simulink model "ReservoirMPC"  (R2023a)
settings: Solver=VariableStepAuto  StartTime=0.0  StopTime=100.0  RelTol=1e-3
libraries: mpclib x1
settings Model: Creator=The MathWorks, Inc.  LastModifiedBy=The MathWorks, Inc.
settings DebuggingCC: UnconnectedInputMsg=warning  UnconnectedOutputMsg=warning  UnconnectedLineMsg=warning
settings ModelReferenceCC: EnableRefExpFcnMdlSchedulingChecks=on
settings RTWCC: DLArmComputeVersion=19.05

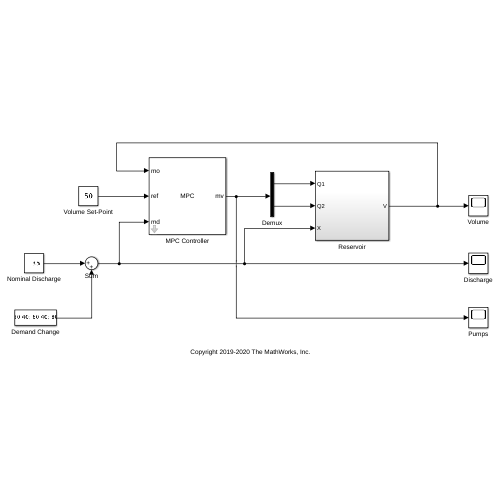
[thumbnail: Simulink's stored preview of the top-level diagram]
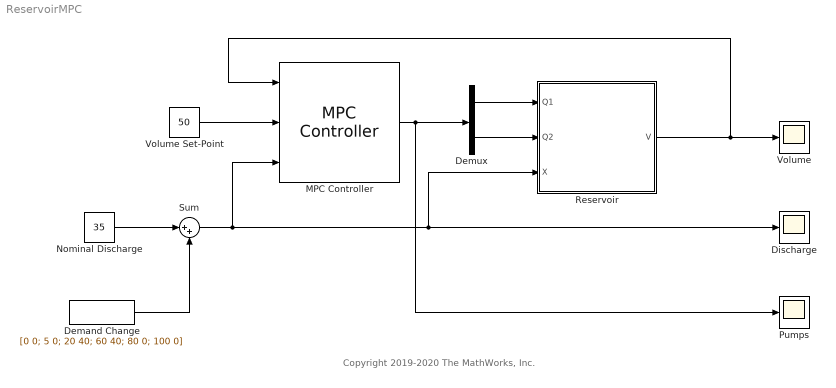
== system ReservoirMPC ==
  note: Copyright 2019-2020 The MathWorks, Inc.
  Demand Change : FromWorkspace  VariableName=[0 0; 5 0; 20 40; 60 40; 80 0; 100 0]
  Demux : Demux  Outputs=2
  Discharge : Scope
  MPC Controller : mpclib/MPC Controller  SCDEnableBlockLinearizationSpecification=on  mpcobj=mpcobj  is_multiple=0  enable_value=0  return_u0=off  updateMPCinCallerWorkspace=on  md_inport=on  mv_inport=off  uref_inport=off  return_cost=off  return_mvseq=off  return_qpstatus=off  return_xseq=off  return_state=off  return_ovseq=off  state_inport=off  umin_inport=off  umax_inport=off  ymin_inport=off  ymax_inport=off  cc_inport=off  ywt_inport=off  uwt_inport=off  duwt_inport=off  rhoeps_inport=off  pm_inport=off  MaximumP=10  HorizonChoice=FixedHorizon  n_ts=1  n_p=10  n_mv=2  n_md=1  n_ud=0  n_mo=1  n_uo=0  BlockDataType=double  SampleTimeInherited=off  switch_inport=off
  Nominal Discharge : Constant  Value=35
  Pumps : Scope
  Reservoir : Subsystem
  Sum : Sum  Inputs=|++
  Volume : Scope
  Volume Set-Point : Constant  Value=50
  wires:
  Reservoir/1(V) -> MPC Controller/1, Volume/1
  Demux/1 -> Reservoir/1(Q1)
  Demux/2 -> Reservoir/2(Q2)
  MPC Controller/1 -> Demux/1, Pumps/1
  Volume Set-Point/1 -> MPC Controller/2
  Nominal Discharge/1 -> Sum/1
  Demand Change/1 -> Sum/2
  Sum/1 -> Reservoir/3(X), Discharge/1, MPC Controller/3

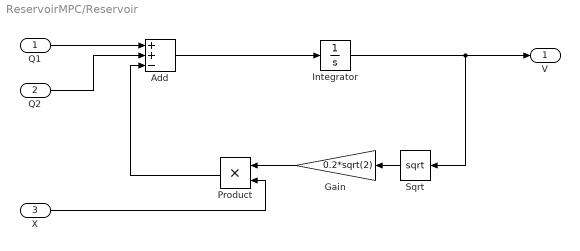
== system ReservoirMPC/Reservoir ==
  Q1 : Inport
  Q2 : Inport  Port=2
  X : Inport  Port=3
  Add : Sum  Inputs=++-
  Gain : Gain  Gain=0.2*sqrt(2)
  Integrator : Integrator  InitialCondition=50  LimitOutput=on  UpperSaturationLimit=100  LowerSaturationLimit=0
  Product : Product
  Sqrt : Sqrt
  V : Outport
  wires:
  X/1 -> Product/2
  Product/1 -> Add/3
  Q2/1 -> Add/2
  Add/1 -> Integrator/1
  Gain/1 -> Product/1
  Q1/1 -> Add/1
  Sqrt/1 -> Gain/1
  Integrator/1 -> Sqrt/1, V/1
